simulink model "Project_2_2_3"  (R2016b)
settings: Solver=VariableStepAuto  StartTime=0.0  StopTime=2  RelTol=1e-3
values from neighbouring files (symbols this model uses):
  A = [A_zero I; -inv(M)*K -inv(M)*D]    [Final_Project_JustinGarcia.m]    (also in Final_Project_Justin_Garcia_190.m = [A_zero initial; -inv(M)*K_equation -inv(M)*D]; projectpart1.m = [zeros(2,2) [1 0;0 1] ; -inv(M)*K -inv(M)*D])
  B = [B_zero;inv(M)*F]    [Final_Project_JustinGarcia.m]    (also in Final_Project_Justin_Garcia_190.m; projectpart1.m = [zeros(2,1); inv(M)*F])
  initial = [0;(4*pi)/180;0;0]    [Final_Project_Justin_Garcia_190.m]
  K_acker = Klqr    [Final_Project_Justin_Garcia_190.m]
settings Model: Creator=Mac  LastModifiedBy=Mac

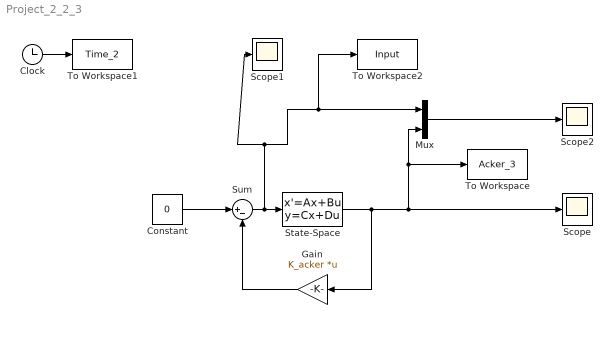
== system Project_2_2_3 ==
  Clock : Clock
  Constant : Constant  Value=0
  Gain : Gain  Gain=K_acker  Multiplication=Matrix(K*u)
  Mux : Mux  Inputs=2
  Scope : Scope
  Scope1 : Scope
  Scope2 : Scope
  State-Space : StateSpace  A=A  B=B  C=[1 0 0 0;0 1 0 0; 0 0 1 0; 0 0 0 1]  D=[0;0;0;0]  X0=initial
  Sum : Sum  Inputs=|+-
  To Workspace : ToWorkspace  VariableName=Acker_3  SampleTime=-1
  To Workspace1 : ToWorkspace  VariableName=Time_2  SampleTime=-1
  To Workspace2 : ToWorkspace  VariableName=Input  SampleTime=-1
  wires:
  Constant/1 -> Sum/1
  State-Space/1 -> Gain/1, To Workspace/1, Mux/2, Scope/1
  Gain/1 -> Sum/2
  Sum/1 -> To Workspace2/1, Mux/1, Scope1/1, State-Space/1
  Mux/1 -> Scope2/1
  Clock/1 -> To Workspace1/1
